simulink model "dynamicModel"  (R2024a)
settings: Solver=ode15s  StartTime=0.0  StopTime=Inf  MaxStep=0.2  RelTol=1e-4
PostLoadFcn:
  | mdlPostLoadFx;
values from neighbouring files (symbols this model uses):
  A = dACpipe.^2.*pi./4    [loadGeometry.m]
  baffleCorr = baffleMat(i,:)    [baffleCalib.m]    (also in calcStatic.m; getBCF.m; mdlPostLoadFx.m = ones(1,3))
  c = getConstants()    [calcPartDisp.m]    (also in getConstants.m = struct(); mdlPostLoadFx.m = 19317.8340012; prepStatic.m)
  d_p = 174.494e-6    (= 0.000174494)    [loadGeometry.m]
  deltaX = 20e-3    (= 0.02)    [loadGeometry.m]
  eps2 = 1.10169319091282    (= 1.10169319091)    [mdlPostLoadFx.m]
  eps3 = -2.04940397390448    (= -2.0494039739)    [mdlPostLoadFx.m]
  epsAr = 0.108571357573225    (= 0.108571357573)    [mdlPostLoadFx.m]
  HAC = mAC.*DryAir.h(TAC)    [getBIC.m]
  href = 1    [loadGeometry.m]
  hTotal = 1.4715    [loadGeometry.m]
  isStatic = false    [mdlPostLoadFx.m]
  Kvs = Kvs.*(1/60^2*sqrt(1000/0.1e6))    [loadGeometry.m]
  l = 0.5    [loadGeometry.m]
  mAB = p0.*VABs./(DryAir.R.*TAB)    [getBIC.m]
  mAC = VAC.*DryAir.rho(p0,TAC)    [getBIC.m]
  maxSimTime = 600    [mdlPostLoadFx.m]
  mDotSstatic = getMdotSstatic(flow.mDotS,direction)    [mdlPostLoadFx.m]
  minSimTime = 240    [mdlPostLoadFx.m]
  n = length(left)    [getBIC.m]    (also in loadGeometry.m = round(sum(xChambers)./deltaX))
  nABs = length(xChambers)    [loadGeometry.m]
  nACs = nABs-2    [loadGeometry.m]
  p0 = flow.p0(i)    [baffleCalib.m]    (also in calcStatic.m; getBCF.m; getBIC.m = flow.p0; mdlPostLoadFx.m = flow.p0(1))
  Phi = h./href.*rho_p.*(1-poro{1,1})    [getBIC.m]
  Phigate = flow.Phigate(i)    [baffleCalib.m]    (also in calcStatic.m; getBCF.m; mdlPostLoadFx.m = hGate./href.*rho_p.*(1-flow.epsRight(1))+p0./(FluBed.g.*href)
  posABs = cell2mat(posABcell)    [loadGeometry.m]
  posACs = posABs-1    [loadGeometry.m]
  rho_p = 2650    [loadGeometry.m]
  s = 5e-3    (= 0.005)    [loadGeometry.m]
  SetMan = false    [mdlPostLoadFx.m]
  statCond = 1e-4    (= 0.0001)    [mdlPostLoadFx.m]
  VABs = NaN(1,length(xChambers))    [loadGeometry.m]
  YMan = [1,1]    [mdlPostLoadFx.m]
undefined symbols (not defined in the file or in its folder): DryAir
libraries: slpidlib x1, simulink x1, slctrl_utilities x1
settings Model: PacingRate=0.500000  Creator=sthanhe  LastModifiedBy=sthanhe
settings SolverCC: MinimalZcImpactIntegration=on
settings DataIOCC: ExternalInput=bc  InitialState=xInit  LoadExternalInput=on  SaveFinalState=on  SaveOutput=off  SignalLogging=off  DSMLogging=off
settings DebuggingCC: ReadBeforeWriteMsg=DisableAll  WriteAfterWriteMsg=DisableAll  WriteAfterReadMsg=DisableAll  AlgebraicLoopMsg=none  MultiTaskDSMMsg=none
settings ModelReferenceCC: UpdateModelReferenceTargets=IfOutOfDate
settings SFSimCC: SFSimEcho=off
settings RTWCC: GPUComputeCapability=3.5

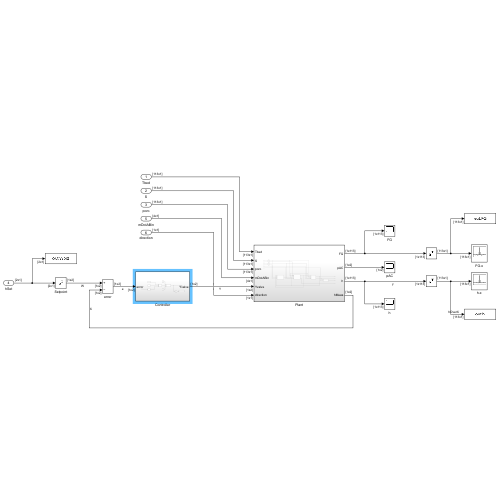
[thumbnail: Simulink's stored preview of the top-level diagram]
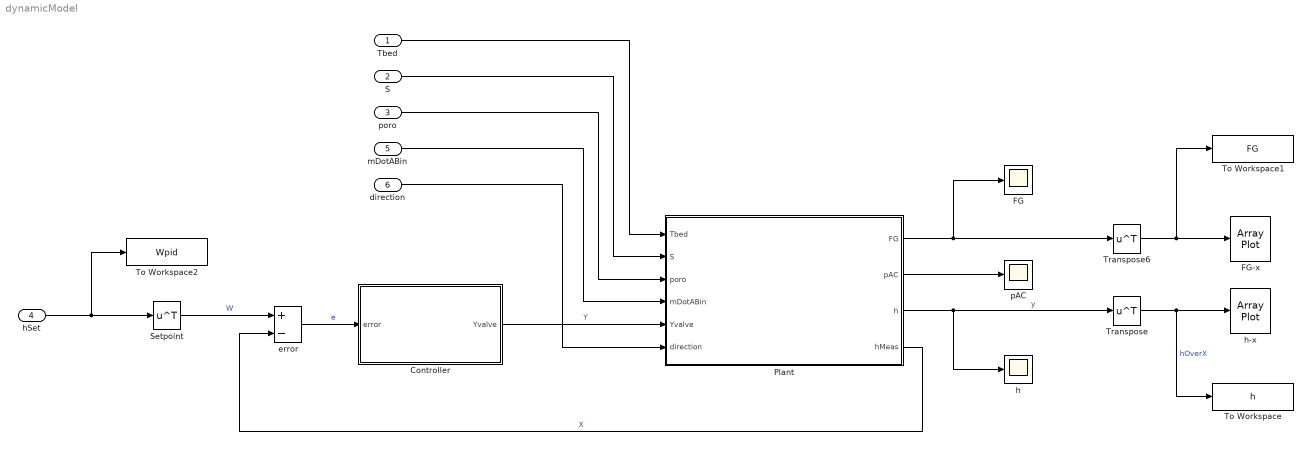
== system dynamicModel ==
  Tbed : Inport  OutDataTypeStr=double  Unit=K  PortDimensions=[n,1]  SampleTime=0
  S : Inport  Port=2  OutDataTypeStr=double  Unit=kg/m^3/s  PortDimensions=[n,1]  SampleTime=0
  poro : Inport  Port=3  OutDataTypeStr=double  Unit=1  PortDimensions=[n,1]  SampleTime=0
  hSet : Inport  Port=4  OutDataTypeStr=double  Unit=m  PortDimensions=[nACs,1]  SampleTime=0
  mDotABin : Inport  Port=5  OutDataTypeStr=double  Unit=kg/s  PortDimensions=[nABs,1]  SampleTime=0
  direction : Inport  Port=6  OutDataTypeStr=double  Unit=1  PortDimensions=[1,1]
  Controller : Subsystem
  FG : Scope
  FG-x : ArrayPlot  WindowPosition=[770.000000,31.000000,766.000000,385.000000,]  ScopeFrameLocation=window  SampleIncrement=deltaX  PlotType=Line  AxesScaling=Auto  YLimits=[1.108 2.5919]
      settings: OpenAtSimulationStart=off
  Plant : Subsystem
  Setpoint : Math  Operator=transpose
  To Workspace : ToWorkspace  VariableName=h  SaveFormat=Timeseries  SampleTime=-1
  To Workspace1 : ToWorkspace  VariableName=FG  SaveFormat=Timeseries  SampleTime=-1
  To Workspace2 : ToWorkspace  VariableName=Wpid  SaveFormat=Timeseries  SampleTime=-1
  Transpose : Math  Operator=transpose
  Transpose6 : Math  Operator=transpose
  error : Sum  Inputs=+-
  h : Scope
  h-x : ArrayPlot  WindowPosition=[385.000000,240.000000,766.000000,385.000000,]  ScopeFrameLocation=window  SampleIncrement=deltaX  PlotType=Line  AxesScaling=Auto  YLimits=[0.4003 0.5422]
      settings: OpenAtSimulationStart=off
  pAC : Scope
  wires:
  S/1 -> Plant/2(S)
  Plant/1(FG) -> Transpose6/1, FG/1
  Tbed/1 -> Plant/1(Tbed)
  Plant/2(pAC) -> pAC/1
  Transpose/1 -> To Workspace/1, h-x/1  "hOverX"
  mDotABin/1 -> Plant/4(mDotABin)
  Transpose6/1 -> To Workspace1/1, FG-x/1
  Plant/3(h) -> Transpose/1, h/1  "y"
  poro/1 -> Plant/3(poro)
  Controller/1(Yvalve) -> Plant/5(Yvalve)  "Y"
  hSet/1 -> Setpoint/1, To Workspace2/1
  error/1 -> Controller/1(error)  "e"
  Plant/4(hMeas) -> error/2  "X"
  Setpoint/1 -> error/1  "W"
  direction/1 -> Plant/6(direction)

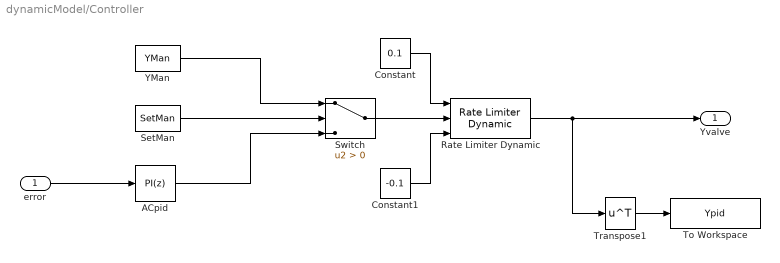
== system dynamicModel/Controller ==
  error : Inport
  ACpid : slpidlib/PID Controller  Controller=PI  Form=Parallel  TimeDomain=Discrete-time  UseExternalTs=off  SampleTime=0.1  IntegratorMethod=Forward Euler  FilterMethod=Forward Euler  ControllerParametersSource=internal  P=10  I=0.1  UseKiTs=on  D=0  UseExternalDerivativeSource=off  N=100  UseFilter=on  TunerSelectOption=Transfer Function Based (PID Tuner App)  InitialConditionSource=internal  InitialConditionForIntegrator=Y0  InitialConditionForFilter=0  DifferentiatorICPrevScaledInput=0  ExternalReset=none  TrackingMode=off  Kt=1  LimitOutput=on  SatLimitsSource=internal  UpperSaturationLimit=0.6  LowerSaturationLimit=0  LinearizeAsGain=on  AntiWindupMode=clamping  Kb=1  LimitIntegrator=off  UpperIntegratorSaturationLimit=inf  LowerIntegratorSaturationLimit=-inf  POutMin=[]  POutMax=[]  IOutMin=[]  IOutMax=[]  DOutMin=[]  DOutMax=[]  NOutMin=[]  NOutMax=[]  SumOutMin=[]  SumOutMax=[]  SaturationOutMin=[]  SaturationOutMax=[]  PParamMin=[]  PParamMax=[]  IParamMin=[]  IParamMax=[]  DParamMin=[]  DParamMax=[]  NParamMin=[]  NParamMax=[]  KbParamMin=[]  KbParamMax=[]  KtParamMin=[]  KtParamMax=[]  KbOutMin=[]  KbOutMax=[]  KtOutMin=[]  KtOutMax=[]  IntegratorOutMin=[]  IntegratorOutMax=[]  FilterOutMin=[]  FilterOutMax=[]  SumI1OutMin=[]  SumI1OutMax=[]  SumI2OutMin=[]  SumI2OutMax=[]  SumI3OutMin=[]  SumI3OutMax=[]  SumI4OutMin=[]  SumI4OutMax=[]  SumDOutMin=[]  SumDOutMax=[]  DifferentiatorOutMin=[]  DifferentiatorOutMax=[]  FilterDiffOutCoefMin=[]  FilterDiffOutCoefMax=[]  ReciprocalOutMin=[]  ReciprocalOutMax=[]  SumDenOutMin=[]  SumDenOutMax=[]  SumNumOutMin=[]  SumNumOutMax=[]  DivideOutMin=[]  DivideOutMax=[]  UdiffTsProdOutMin=[]  UdiffTsProdOutMax=[]  NTsProdOutMin=[]  NTsProdOutMax=[]  UintegralTsProdOutMin=[]  UintegralTsProdOutMax=[]  UngainTsProdOutMin=[]  UngainTsProdOutMax=[]  ClampingZeroOutDataTypeStr=Inherit: Inherit via back propagation  ClampingZeroOutMin=[]  ClampingZeroOutMax=[]  FilterDenConstantOutDataTypeStr=Inherit: Inherit via back propagation  FilterDenConstantOutMin=[]  FilterDenConstantOutMax=[]  PCopyOutDataTypeStr=Inherit: Inherit via back propagation  PCopyOutMin=[]  PCopyOutMax=[]  NCopyOutDataTypeStr=Inherit: Inherit via back propagation  NCopyOutMin=[]  NCopyOutMax=[]  IntegratorContinuousStateAttributes='AC'  IntegratorStateIdentifier=ACpid  IntegratorStateMustResolveToSignalObject=off  IntegratorRTWStateStorageClass=Auto  FilterContinuousStateAttributes=''  FilterStateMustResolveToSignalObject=off  FilterRTWStateStorageClass=Auto  ParallelPVariant=InternalParameters  IdealPVariant=Disabled  IVariant=InternalParameters  DVariant=Disabled  IntegratorVariant=Discrete  SatVariant=Enabled  AWVariant=DiscClampingParallel  PCopyVariant=Disabled  TRVariant=Disabled  FdbkBlocksVariant=Forward  IdealPFdbkVariant=Disabled  SatFdbkVariant=Disabled  DerivativeFilterVariant=Disabled  NVariant=Disabled  NCopyVariant=Disabled_SignalSpec  FilterICVariant=Disabled  IntegratorICVariant=InternalICs  ExternalResetVariant=Disabled  TRSumVariant=Passthrough  SumFdbkVariant=Disabled  SumVariant=Sum_PI  TsampFilterVariant=InternalTs  TsampNgainVariant=Passthrough  TsampIntegralVariant=Disabled_SignalSpec  ExternalSaturationOutDataTypeStr=Inherit: Same as second input  DerivativeSourceVariant=Disabled
  Constant : Constant  Value=0.1
  Constant1 : Constant  Value=-0.1
  Rate Limiter Dynamic : simulink/Discontinuities/Rate Limiter Dynamic
  SetMan : Constant  Value=SetMan
  Switch : Switch  Criteria=u2 > Threshold  SaturateOnIntegerOverflow=off  InputSameDT=off
  To Workspace : ToWorkspace  VariableName=Ypid  SaveFormat=Timeseries  SampleTime=-1
  Transpose1 : Math  Operator=transpose
  YMan : Constant  Value=YMan
  Yvalve : Outport
  wires:
  Transpose1/1 -> To Workspace/1
  Rate Limiter Dynamic/1 -> Yvalve/1, Transpose1/1
  error/1 -> ACpid/1
  ACpid/1 -> Switch/3
  SetMan/1 -> Switch/2
  YMan/1 -> Switch/1
  Switch/1 -> Rate Limiter Dynamic/2
  Constant/1 -> Rate Limiter Dynamic/1
  Constant1/1 -> Rate Limiter Dynamic/3

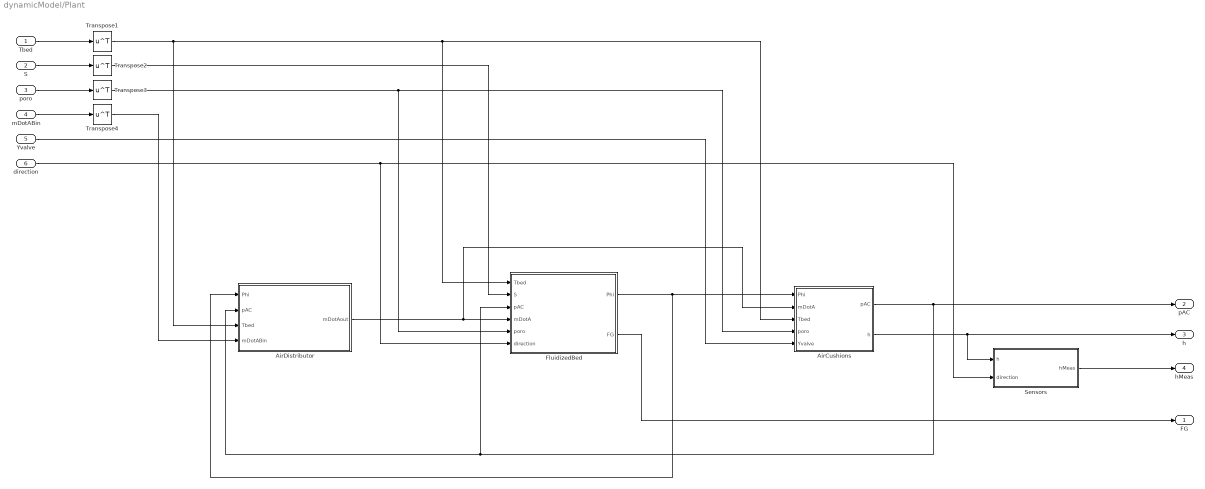
== system dynamicModel/Plant ==
  Tbed : Inport  OutDataTypeStr=double  Unit=K  PortDimensions=[n,1]  SampleTime=0
  S : Inport  Port=2  OutDataTypeStr=double  Unit=kg/m^3/s  PortDimensions=[n,1]  SampleTime=0
  poro : Inport  Port=3  OutDataTypeStr=double  Unit=1  PortDimensions=[n,1]  SampleTime=0
  mDotABin : Inport  Port=4  OutDataTypeStr=double  Unit=kg/s  PortDimensions=[nABs,1]  SampleTime=0
  Yvalve : Inport  Port=5
  direction : Inport  Port=6
  AirCushions : Subsystem
  AirDistributor : Subsystem
  FluidizedBed : Subsystem
  Sensors : Subsystem
  Transpose{1..4} (4 alike) : Math  Operator=transpose
  FG : Outport
  pAC : Outport  Port=2
  h : Outport  Port=3
  hMeas : Outport  Port=4
  wires:
  AirCushions/1(pAC) -> FluidizedBed/3(pAC), AirDistributor/2(pAC), pAC/1
  Tbed/1 -> Transpose1/1
  Transpose1/1 -> AirCushions/3(Tbed), FluidizedBed/1(Tbed), AirDistributor/3(Tbed)
  mDotABin/1 -> Transpose4/1
  AirDistributor/1(mDotAout) -> AirCushions/2(mDotA), FluidizedBed/4(mDotA)
  FluidizedBed/1(Phi) -> AirDistributor/1(Phi), AirCushions/1(Phi)
  FluidizedBed/2(FG) -> FG/1
  poro/1 -> Transpose3/1
  Transpose2/1 -> FluidizedBed/2(S)
  S/1 -> Transpose2/1
  Transpose3/1 -> AirCushions/4(poro), FluidizedBed/5(poro)
  AirCushions/2(h) -> Sensors/1(h), h/1
  Transpose4/1 -> AirDistributor/4(mDotABin)
  Yvalve/1 -> AirCushions/5(Yvalve)
  direction/1 -> FluidizedBed/6(direction), Sensors/2(direction)
  Sensors/1(hMeas) -> hMeas/1

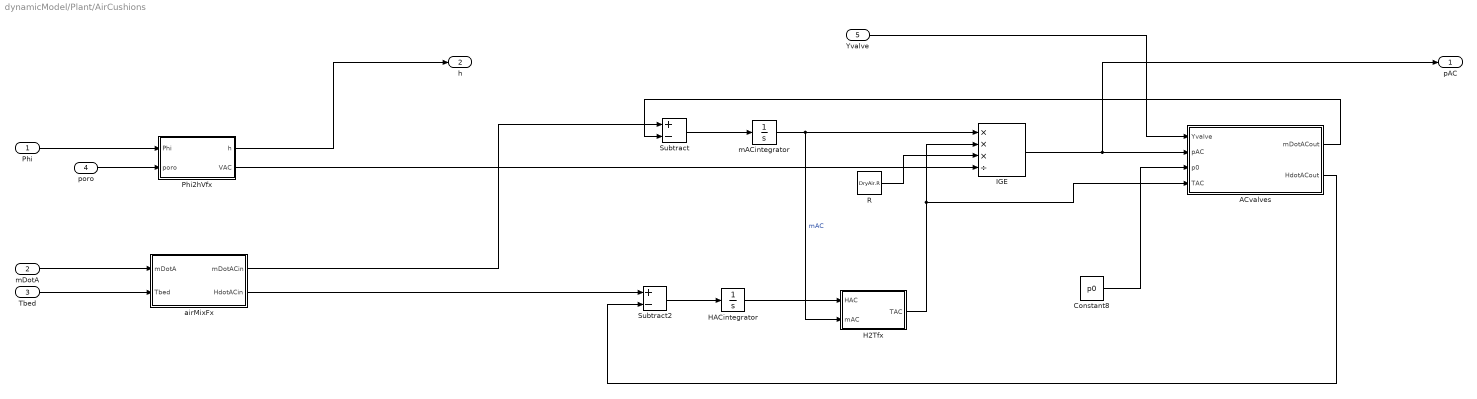
== system dynamicModel/Plant/AirCushions ==
  Phi : Inport
  mDotA : Inport  Port=2
  Tbed : Inport  Port=3
  poro : Inport  Port=4
  Yvalve : Inport  Port=5
  ACvalves : MATLAB Function  TreatAsAtomicUnit=on
  Constant8 : Constant  Value=p0
  H2Tfx : MATLAB Function  TreatAsAtomicUnit=on
  HACintegrator : Integrator  InitialCondition=HAC  ContinuousStateAttributes='HAC'
  IGE : Product  Inputs=***/
  Phi2hVfx : MATLAB Function  TreatAsAtomicUnit=on
  R : Constant  Value=DryAir.R
  Subtract : Sum  Inputs=+-
  Subtract2 : Sum  Inputs=+-
  airMixFx : MATLAB Function  TreatAsAtomicUnit=on
  mACintegrator : Integrator  InitialCondition=mAC  LowerSaturationLimit=0  ContinuousStateAttributes='mAC'
  pAC : Outport
  h : Outport  Port=2
  wires:
  R/1 -> IGE/3
  Subtract/1 -> mACintegrator/1
  airMixFx/1(mDotACin) -> Subtract/1
  Constant8/1 -> ACvalves/3(p0)
  Tbed/1 -> airMixFx/2(Tbed)
  Phi2hVfx/2(VAC) -> IGE/4
  H2Tfx/1(TAC) -> IGE/2, ACvalves/4(TAC)
  mDotA/1 -> airMixFx/1(mDotA)
  mACintegrator/1 -> IGE/1, H2Tfx/2(mAC)  "mAC"
  ACvalves/1(mDotACout) -> Subtract/2
  ACvalves/2(HdotACout) -> Subtract2/2
  Subtract2/1 -> HACintegrator/1
  airMixFx/2(HdotACin) -> Subtract2/1
  HACintegrator/1 -> H2Tfx/1(HAC)
  IGE/1 -> pAC/1, ACvalves/2(pAC)
  Phi/1 -> Phi2hVfx/1(Phi)
  poro/1 -> Phi2hVfx/2(poro)
  Phi2hVfx/1(h) -> h/1
  Yvalve/1 -> ACvalves/1(Yvalve)

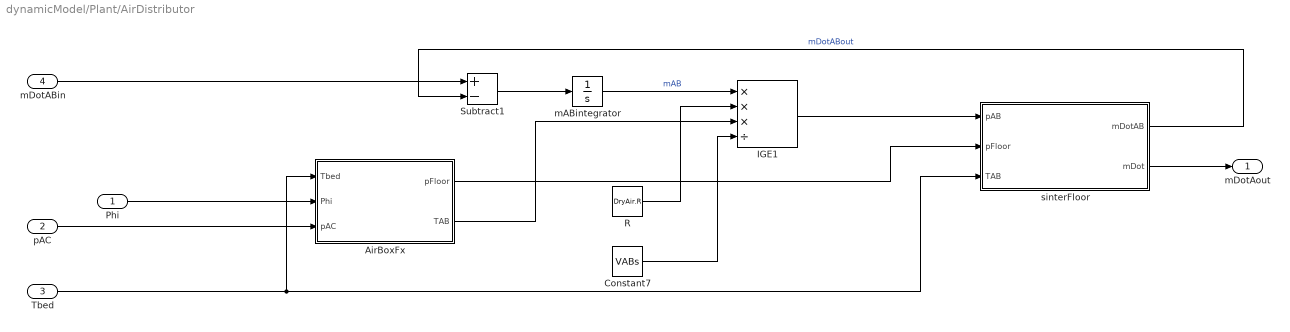
== system dynamicModel/Plant/AirDistributor ==
  Phi : Inport
  pAC : Inport  Port=2
  Tbed : Inport  Port=3
  mDotABin : Inport  Port=4
  AirBoxFx : MATLAB Function  TreatAsAtomicUnit=on
  Constant7 : Constant  Value=VABs
  IGE1 : Product  Inputs=***/
  R : Constant  Value=DryAir.R
  Subtract1 : Sum  Inputs=+-
  mABintegrator : Integrator  InitialCondition=mAB  ContinuousStateAttributes='mAB'
  sinterFloor : MATLAB Function  TreatAsAtomicUnit=on
  mDotAout : Outport
  wires:
  pAC/1 -> AirBoxFx/3(pAC)
  Tbed/1 -> AirBoxFx/1(Tbed), sinterFloor/3(TAB)
  AirBoxFx/2(TAB) -> IGE1/3
  R/1 -> IGE1/2
  mDotABin/1 -> Subtract1/1
  sinterFloor/1(mDotAB) -> Subtract1/2  "mDotABout"
  Constant7/1 -> IGE1/4
  Subtract1/1 -> mABintegrator/1
  Phi/1 -> AirBoxFx/2(Phi)
  IGE1/1 -> sinterFloor/1(pAB)
  AirBoxFx/1(pFloor) -> sinterFloor/2(pFloor)
  mABintegrator/1 -> IGE1/1  "mAB"
  sinterFloor/2(mDot) -> mDotAout/1

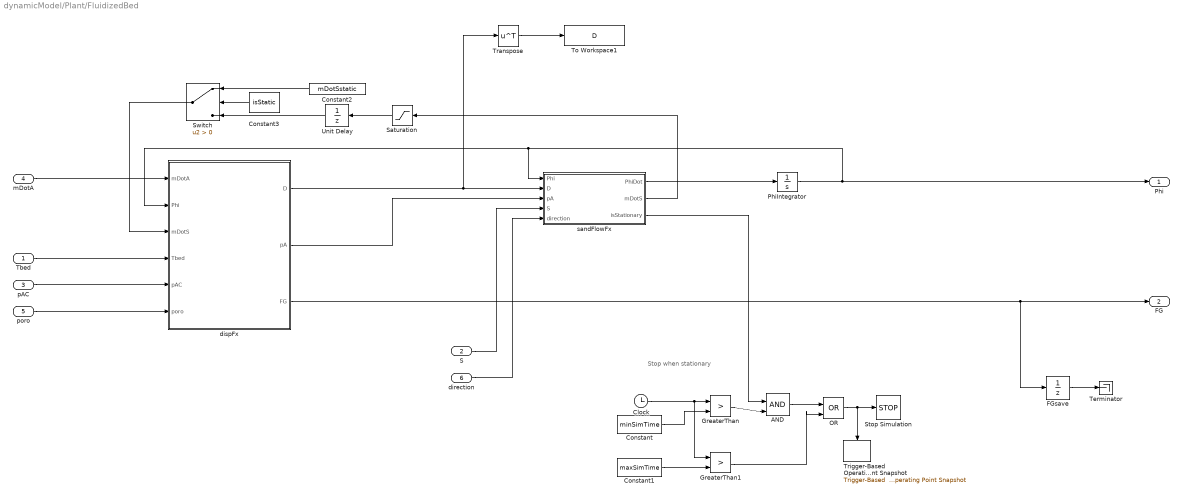
== system dynamicModel/Plant/FluidizedBed ==
  note: Stop when stationary
  Tbed : Inport
  S : Inport  Port=2
  pAC : Inport  Port=3
  mDotA : Inport  Port=4
  poro : Inport  Port=5
  direction : Inport  Port=6
  AND : Logic  IconShape=distinctive  AllPortsSameDT=off  OutDataTypeStr=boolean
  Clock : Clock
  Constant : Constant  Value=minSimTime
  Constant1 : Constant  Value=maxSimTime
  Constant2 : Constant  Value=mDotSstatic
  Constant3 : Constant  Value=isStatic
  FGsave : UnitDelay  SampleTime=-1  StateName=FGsave  HasFrameUpgradeWarning=on
  GreaterThan : RelationalOperator  Operator=>  OutDataTypeStr=boolean  RndMeth=Simplest  InputSameDT=off
  GreaterThan1 : RelationalOperator  Operator=>  OutDataTypeStr=boolean  RndMeth=Simplest  InputSameDT=off
  OR : Logic  Operator=OR  IconShape=distinctive  AllPortsSameDT=off  OutDataTypeStr=boolean
  PhiIntegrator : Integrator  InitialCondition=Phi  ContinuousStateAttributes='Phi'
  Saturation : Saturate  UpperLimit=12  LowerLimit=-12  ZeroCross=off  OutDataTypeStr=double
  Stop Simulation : Stop
  Switch : Switch  Criteria=u2 > Threshold  SaturateOnIntegerOverflow=off  InputSameDT=off
  Terminator : Terminator
  To Workspace1 : ToWorkspace  VariableName=D  SaveFormat=Timeseries  SampleTime=-1
  Transpose : Math  Operator=transpose
  Trigger-Based Operating Point Snapshot : slctrl_utilities/Trigger-Based  Operating Point Snapshot  TriggerType=rising
      settings: LibrarySourceBlock=|
      | slctrlblks/Utilities/Trigger-Based
      | Operating Point
      | Snapshot
  Unit Delay : UnitDelay  InitialCondition=mDotSstatic  SampleTime=-1  StateName=mDotS  HasFrameUpgradeWarning=on
  dispFx : MATLAB Function  TreatAsAtomicUnit=on
  sandFlowFx : MATLAB Function  TreatAsAtomicUnit=on
  Phi : Outport
  FG : Outport  Port=2
  wires:
  Tbed/1 -> dispFx/4(Tbed)
  mDotA/1 -> dispFx/1(mDotA)
  sandFlowFx/1(PhiDot) -> PhiIntegrator/1
  S/1 -> sandFlowFx/4(S)
  pAC/1 -> dispFx/5(pAC)
  direction/1 -> sandFlowFx/5(direction)
  dispFx/2(pA) -> sandFlowFx/3(pA)
  PhiIntegrator/1 -> dispFx/2(Phi), sandFlowFx/1(Phi), Phi/1
  Transpose/1 -> To Workspace1/1
  Clock/1 -> GreaterThan/1, GreaterThan1/1
  Constant/1 -> GreaterThan/2
  GreaterThan/1 -> AND/2
  sandFlowFx/3(isStationary) -> AND/1
  AND/1 -> OR/1
  OR/1 -> Stop Simulation/1, Trigger-Based Operating Point Snapshot/Trigger
  GreaterThan1/1 -> OR/2
  Constant1/1 -> GreaterThan1/2
  poro/1 -> dispFx/6(poro)
  Saturation/1 -> Unit Delay/1
  sandFlowFx/2(mDotS) -> Saturation/1
  dispFx/1(D) -> Transpose/1, sandFlowFx/2(D)
  Switch/1 -> dispFx/3(mDotS)
  Unit Delay/1 -> Switch/3
  Constant3/1 -> Switch/2
  Constant2/1 -> Switch/1
  dispFx/3(FG) -> FGsave/1, FG/1
  FGsave/1 -> Terminator/1

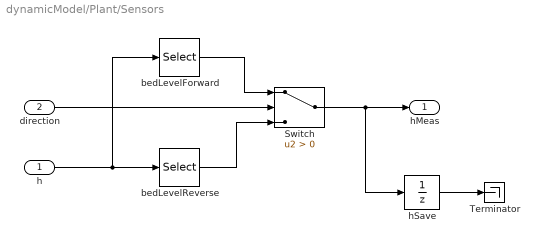
== system dynamicModel/Plant/Sensors ==
  h : Inport
  direction : Inport  Port=2
  Switch : Switch  Criteria=u2 > Threshold  SaturateOnIntegerOverflow=off  InputSameDT=off
  Terminator : Terminator
  bedLevelForward : Selector  InputPortWidth=n  IndexOptions=Index vector (dialog)  Indices=posBedLevelForward  OutputSizes=1
  bedLevelReverse : Selector  InputPortWidth=n  IndexOptions=Index vector (dialog)  Indices=posBedLevelReverse  OutputSizes=1
  hSave : UnitDelay  SampleTime=-1  StateName=hSave  HasFrameUpgradeWarning=on
  hMeas : Outport
  wires:
  h/1 -> bedLevelForward/1, bedLevelReverse/1
  bedLevelReverse/1 -> Switch/3
  bedLevelForward/1 -> Switch/1
  direction/1 -> Switch/2
  Switch/1 -> hMeas/1, hSave/1
  hSave/1 -> Terminator/1

== matlab function dynamicModel/Plant/AirCushions/airMixFx ==
  data: mDotACin output; mDotA input double size=[1,n]; HdotACin output double size=[1,nACs]; Tbed input double size=[1,n]; nACs parameter double size=1; posACs parameter double size=[1,n]
function [mDotACin,HdotACin]=airMix(mDotA,Tbed,nACs,posACs)
    %Aggregate cell air mass flows to air cushions
    mDotACin=arrayfun(@(x) sum(mDotA(posACs==x)),1:nACs);

    %Get total enthalpy flows per air cushion
    HdotACin=arrayfun(@(x) sum(mDotA(posACs==x).*DryAir.h(Tbed(posACs==x))),1:nACs);
end

== matlab function dynamicModel/Plant/AirCushions/H2Tfx ==
  data: HAC input double size=[1,nACs]; TAC output double size=[1,nACs]; mAC input double size=[1,nACs]
function TAC=H2T(HAC,mAC)
    %Get specific air temperature from its enthalpy
    TAC=DryAir.T_h(HAC./mAC);
end

== matlab function dynamicModel/Plant/AirDistributor/AirBoxFx ==
  data: Tbed input double size=[1,n]; pFloor output double size=[1,n]; Phi input double size=[1,n]; pAC input double size=[1,nACs]; p0 parameter double size=1; posACs parameter size=[1,n]; posABs parameter double size=[1,n]; nABs parameter double size=1; TAB output double size=[1,nABs]; href parameter double size=1
function [pFloor,TAB]=ABvalues(Tbed,Phi,pAC,p0,posACs,posABs,nABs,href)
    %Assign air cushion pressure to cells
    pAC=[p0,pAC];
    pA=pAC(posACs+1);

    %Calculate pressure above floor
    pFloor=pA+Phi.*FluBed.g.*href;
    
    %Assume the temperature in the air box to be the mean of the bed
    %temperature above it
    TAB=arrayfun(@(x) mean(Tbed(posABs==x)),1:nABs);
end

== matlab function dynamicModel/Plant/AirCushions/Phi2hVfx ==
  data: Phi input double size=[1,n]; poro input double size=[1,n]; h output double size=[1,n]; href parameter double size=1; hTotal parameter size=1; rho_p parameter double size=1; VAC output size=[1,nACs]; posACs parameter size=[1,n]; nACs parameter size=1; l parameter size=1; deltaX parameter size=1
function [h,VAC]=Phi2hV(Phi,poro,href,hTotal,rho_p,posACs,nACs,l,deltaX)
    %Get bed levels from density and porosity
    h=Phi.*href./(rho_p.*(1-poro));

    %Calculate air cushion volumes based on bed levels
    Vvec=(hTotal-h).*l.*deltaX;
    VAC=arrayfun(@(x) sum(Vvec(posACs==x)),1:nACs);
end

== matlab function dynamicModel/Plant/FluidizedBed/dispFx ==
  data: mDotA input double size=[1,n]; Phi input double size=[1,n]; mDotS input double size=[1,n]; Tbed input double size=[1,n]; pAC input double size=[1,nACs]; poro input size=[1,n]; D output double size=[1,n]; href parameter double size=1; d_p parameter double size=1; rho_p parameter double size=1; l parameter double size=1; deltaX parameter double size=1; posACs parameter double size=[1,n]; p0 parameter double size=1; c parameter size=1; pA output double size=[1,n]; FG output double size=[1,n]; eps2 parameter size=1; eps3 parameter size=1; epsAr parameter size=1
function [D,pA,FG]=disp(mDotA,Phi,mDotS,Tbed,pAC,poro,href,d_p,rho_p,l,deltaX,posACs,p0,c,eps2,eps3,epsAr)
    %Assign air cushion pressure to cells
    pAC=[p0,pAC];
    pA=pAC(posACs+1);


    %Calculate fluidization
    pBed=pA+Phi.*FluBed.g.*href./2;                 %Mean bed pressure
    wA=mDotA./(DryAir.rho(pBed,Tbed).*l.*deltaX);   %Air velocity
    FG=wA./FluBed.wmf(d_p,rho_p,pBed,Tbed);         %Degree of fluidization (post processing only)


    %Get particle velocities
    h=Phi.*href./(rho_p.*(1-poro));         %Bed levels
    w_p=mDotS.*href./(rho_p.*(1-poro).*h);


    %Get particle dispersion coefficient
    den=sqrt(d_p.*FluBed.g);

    pi2=(wA-FluBed.wmf(d_p,rho_p,pBed,Tbed))./den;
    pi3=abs(w_p)./den;
    Ar=FluBed.Ar(d_p,rho_p,pBed,Tbed);

    pi2(pi2<0)=0;


    D=c.*d_p.*den.*...
        pi2.^eps2.*...
        (1+pi3).^eps3.*...
        Ar.^epsAr;
    
    
end

== matlab function dynamicModel/Plant/FluidizedBed/sandFlowFx ==
  data: Phi input double size=[1,n]; D input double size=[1,n]; pA input double size=[1,n]; S input double size=[1,n]; direction input double size=[1,1]; PhiDot output double size=[1,n]; deltaX parameter double size=1; href parameter double size=1; Phigate parameter double size=1; posACs parameter double size=[1,n]; baffleCorr parameter double size=[1,3]; mDotS output double size=[1,n]; isStationary output boolean size=[1,1]; statCond parameter double size=[1,1]
function [PhiDot,mDotS,isStationary]=sandFlow(Phi,D,pA,S,direction,deltaX,href,Phigate,posACs,baffleCorr,statCond)
    %Add air cushion pressure to density
    Phi=Phi+pA./(FluBed.g.*href);


    %Include boundary conditions at walls: first derivative of Phi is zero,
    %which is equal to boundary values being equal to first inner values. 
    %Vectors are extended accordingly.
    PhiB=[Phi(1),Phi,Phi(end)];
    DB=[D(1),D,D(end)];


    %Boundary conditions where gate is open: Phi is equal to Phi at the
    %open gate (Phigate), but only when Phigate is smaller than Phi,
    %otherwise a backflow would occur. 
    idx=[1,length(PhiB)];
    dirBool=logical(round(direction));
    gates=[~dirBool,dirBool];      %Open / closed gates based on operating direction
    PhiB(idx(gates & Phigate<PhiB([1,end])))=Phigate;


    %Phi and D across cell borders
    Phi_i=PhiB(2:end-1);
    Phi_iplus1=PhiB(3:end);
    Phi_iminus1=PhiB(1:end-2);

    D_half=movmean(DB,2);
    D_iplus1half=D_half(3:end);
    D_iminus1half=D_half(2:end-1);


    %Baffle correction factors
    baffles=find(diff(posACs)~=0);
    for i=1:length(baffles)
        D_iplus1half(baffles(i))=D_iplus1half(baffles(i))./baffleCorr(i);
        D_iminus1half(baffles(i)+1)=D_iminus1half(baffles(i)+1)./baffleCorr(i);
    end

    
    %Specific mass flows
    mDotSL=-D_iminus1half.*(Phi_i-Phi_iminus1)./deltaX;     %Left, into cells
    mDotSR=-D_iplus1half.*(Phi_iplus1-Phi_i)./deltaX;       %Right, out of cells

    mDotS=mean([mDotSL;mDotSR],1);  %Mean


    %Fictional density derivative
    PhiDot=(mDotSL-mDotSR)./deltaX+S;
    
    
    %Check for stationary status
    if all(abs(PhiDot)<statCond)
        isStationary=true;
    else
        isStationary=false;
    end
    
end

== matlab function dynamicModel/Plant/AirCushions/ACvalves ==
  data: Yvalve input double size=[1,nACs]; mDotACout output double size=[1,nACs]; pAC input double size=[1,nACs]; p0 input double size=1; TAC input double size=[1,nACs]; Kvs parameter double size=1; A parameter double size=1; HdotACout output double size=[1,nACs]
function [mDotACout,HdotACout]=valve(Yvalve,pAC,p0,TAC,Kvs,A)
    %Conditions
    Kv=Yvalve.*Kvs;             %Linear valve flow rate
    zeta=2.*A.^2./Kv.^2;        %Pressure loss coefficient
    rho=DryAir.rho(pAC,TAC);    %Air density (upstream)

    %Flow velocity based on pressure loss characteristic
    wA=sqrt(2.*abs(pAC-p0)./(zeta.*rho));
    wA=sign(pAC-p0).*wA;
    
    %Air mass and enthalpy flows
    mDotACout=wA.*A.*rho;
    HdotACout=mDotACout.*DryAir.h(TAC);
end

== matlab function dynamicModel/Plant/AirDistributor/sinterFloor ==
  data: mDotAB output double size=[1,nABs]; pAB input double size=[1,nABs]; mDot output double size=[1,n]; pFloor input double size=[1,n]; TAB input double size=[1,n]; posABs parameter double size=[1,n]; s parameter double size=1; l parameter double size=1; deltaX parameter double size=1
function [mDotAB,mDot]=sinter(pAB,pFloor,TAB,posABs,s,l,deltaX)
    %Assign air box pressures to cell inlet pressures
    pin=pAB(posABs);
    
    %Get mass flows through sinter plate
    mDotS=zeros(size(pFloor));
    idx=pin-pFloor>0;
    [~,~,mDotS(idx)]=Sinter.w(pin(idx),pFloor(idx),TAB(idx),s,'SIKA-R 15 AX');
    mDot=mDotS.*l.*deltaX;

    %Aggregate cell mass flows to air box mass flows
    mDotAB=arrayfun(@(x) sum(mDot(posABs==x)),1:length(pAB));
end
